simulink model "simulink_group8"  (R2020a)
settings: Solver=FixedStepAuto  StartTime=0.0  StopTime=10.0  FixedStep=1e-3  RelTol=1e-3  EnableMultiTasking=on
undefined symbols (not defined in the file): D0, D1, D10, D11, D12, D13, D2, D3, D4, D5, D6, D7, D8, D9, PTA0, PTA1, PTA2, PTB23, PTB9, PTC16, PTC17, PTC2, PTC3, PTC4, PTD0, PTD1, PTD2, PTD3
libraries: frdmk64flib x14
settings Model: ExtModeTrigDuration=5  Creator=namby  LastModifiedBy=namby
settings OptimizationCC: EnhancedBackFolding=on  PassReuseOutputArgsAs=Individual arguments  ZeroExternalMemoryAtStartup=off  ZeroInternalMemoryAtStartup=off  MaxStackSize=64  OptimizeBlockOrder=speed  DifferentSizesBufferReuse=on  OptimizationCustomize=off  EfficientTunableParamExpr=on
settings DebuggingCC: ParameterTunabilityLossMsg=error
settings HardwareCC: ProdBitPerPointer=32  ProdBitPerSizeT=32  ProdBitPerPtrDiffT=32  ProdLargestAtomicInteger=Long  ProdLargestAtomicFloat=Double  ProdWordSize=32  ProdHWDeviceType=ARM Compatible->ARM Cortex
settings SFSimCC: MATLABDynamicMemAlloc=off
settings RTWCC: SystemTargetFile=ert.tlc  HardwareBoard=NXP FRDM-K64F  TemplateMakefile=ert_default_tmf  Toolchain=GNU Tools for ARM Embedded Processors
settings CodeAppCC: ForceParamTrailComments=on  IgnoreCustomStorageClasses=off  OperatorAnnotations=on  SimulinkDataObjDesc=on  SFDataObjDesc=on  InsertBlockDesc=on

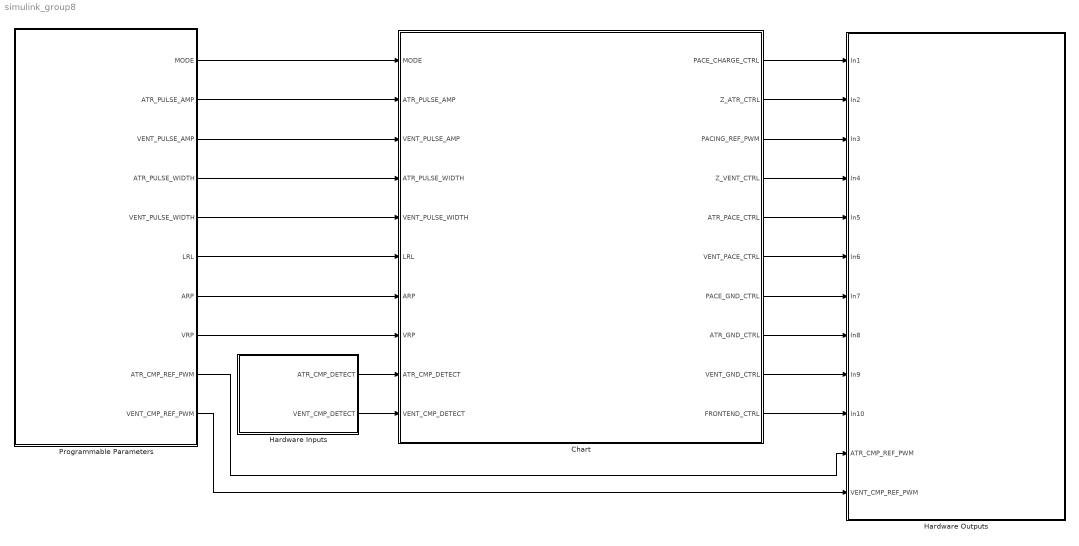
== system simulink_group8 ==
  Chart : Stateflow chart  TreatAsAtomicUnit=on
  Hardware Inputs : Subsystem
  Hardware Outputs : Subsystem
  Programmable Parameters : Subsystem
  wires:
  Programmable Parameters/1(MODE) -> Chart/1(MODE)
  Programmable Parameters/2(ATR_PULSE_AMP) -> Chart/2(ATR_PULSE_AMP)
  Programmable Parameters/3(VENT_PULSE_AMP) -> Chart/3(VENT_PULSE_AMP)
  Programmable Parameters/4(ATR_PULSE_WIDTH) -> Chart/4(ATR_PULSE_WIDTH)
  Programmable Parameters/5(VENT_PULSE_WIDTH) -> Chart/5(VENT_PULSE_WIDTH)
  Programmable Parameters/6(LRL) -> Chart/6(LRL)
  Programmable Parameters/7(ARP) -> Chart/7(ARP)
  Programmable Parameters/8(VRP) -> Chart/8(VRP)
  Hardware Inputs/1(ATR_CMP_DETECT) -> Chart/9(ATR_CMP_DETECT)
  Hardware Inputs/2(VENT_CMP_DETECT) -> Chart/10(VENT_CMP_DETECT)
  Chart/1(PACE_CHARGE_CTRL) -> Hardware Outputs/1(In1)
  Chart/2(Z_ATR_CTRL) -> Hardware Outputs/2(In2)
  Chart/3(PACING_REF_PWM) -> Hardware Outputs/3(In3)
  Chart/4(Z_VENT_CTRL) -> Hardware Outputs/4(In4)
  Chart/5(ATR_PACE_CTRL) -> Hardware Outputs/5(In5)
  Chart/6(VENT_PACE_CTRL) -> Hardware Outputs/6(In6)
  Chart/7(PACE_GND_CTRL) -> Hardware Outputs/7(In7)
  Chart/8(ATR_GND_CTRL) -> Hardware Outputs/8(In8)
  Chart/9(VENT_GND_CTRL) -> Hardware Outputs/9(In9)
  Chart/10(FRONTEND_CTRL) -> Hardware Outputs/10(In10)
  Programmable Parameters/9(ATR_CMP_REF_PWM) -> Hardware Outputs/11(ATR_CMP_REF_PWM)
  Programmable Parameters/10(VENT_CMP_REF_PWM) -> Hardware Outputs/12(VENT_CMP_REF_PWM)

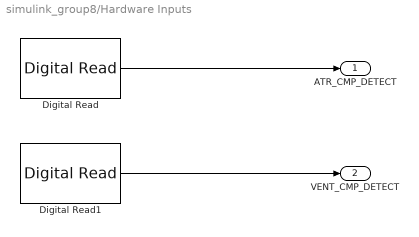
== system simulink_group8/Hardware Inputs ==
  Digital Read : frdmk64flib/Digital Read  Whichpin=PTC16 (D0)  SampleTime=-1
  Digital Read1 : frdmk64flib/Digital Read  Whichpin=PTC17 (D1)  SampleTime=-1
  ATR_CMP_DETECT : Outport
  VENT_CMP_DETECT : Outport  Port=2
  wires:
  Digital Read/1 -> ATR_CMP_DETECT/1
  Digital Read1/1 -> VENT_CMP_DETECT/1

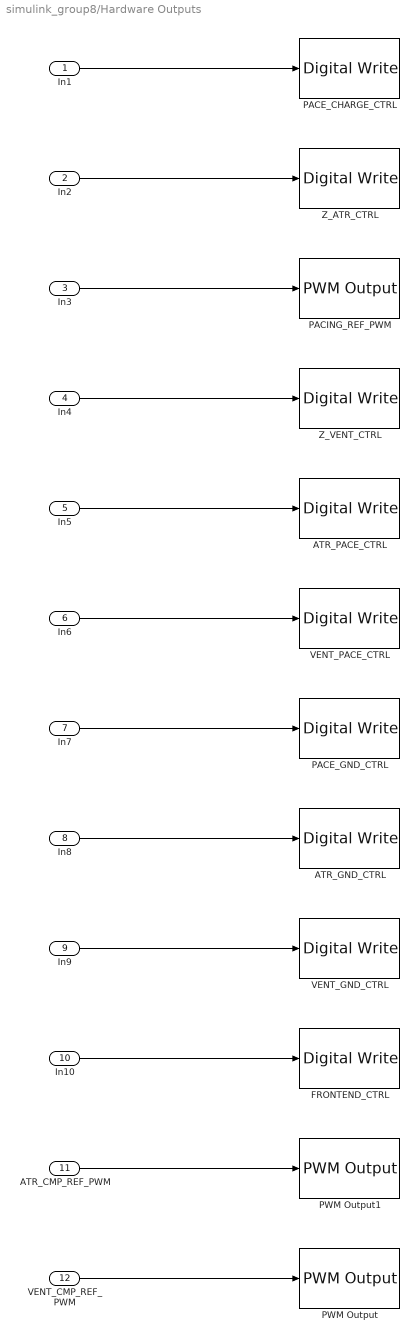
== system simulink_group8/Hardware Outputs ==
  In1 : Inport
  In2 : Inport  Port=2
  In3 : Inport  Port=3
  In4 : Inport  Port=4
  In5 : Inport  Port=5
  In6 : Inport  Port=6
  In7 : Inport  Port=7
  In8 : Inport  Port=8
  In9 : Inport  Port=9
  In10 : Inport  Port=10
  ATR_CMP_REF_PWM : Inport  Port=11
  VENT_CMP_REF_PWM : Inport  Port=12
  ATR_GND_CTRL : frdmk64flib/Digital Write  Whichpin=PTD2 (D11)
  ATR_PACE_CTRL : frdmk64flib/Digital Write  Whichpin=PTA0 (D8)
  FRONTEND_CTRL : frdmk64flib/Digital Write  Whichpin=PTD1 (D13)
  PACE_CHARGE_CTRL : frdmk64flib/Digital Write  Whichpin=PTB9 (D2)
  PACE_GND_CTRL : frdmk64flib/Digital Write  Whichpin=PTD0 (D10)
  PACING_REF_PWM : frdmk64flib/PWM Output  Whichpin=PTA2 (D5)  InitialFrequency=2000  InitialDutyCycle=0
  PWM Output : frdmk64flib/PWM Output  Whichpin=PTA1 (D3)  InitialFrequency=2000  InitialDutyCycle=0
  PWM Output1 : frdmk64flib/PWM Output  Whichpin=PTC2 (D6)  InitialFrequency=2000  InitialDutyCycle=0
  VENT_GND_CTRL : frdmk64flib/Digital Write  Whichpin=PTD3 (D12)
  VENT_PACE_CTRL : frdmk64flib/Digital Write  Whichpin=PTC4 (D9)
  Z_ATR_CTRL : frdmk64flib/Digital Write  Whichpin=PTB23 (D4)
  Z_VENT_CTRL : frdmk64flib/Digital Write  Whichpin=PTC3 (D7)
  wires:
  In1/1 -> PACE_CHARGE_CTRL/1
  In2/1 -> Z_ATR_CTRL/1
  In3/1 -> PACING_REF_PWM/1
  In4/1 -> Z_VENT_CTRL/1
  In5/1 -> ATR_PACE_CTRL/1
  In6/1 -> VENT_PACE_CTRL/1
  In8/1 -> ATR_GND_CTRL/1
  In7/1 -> PACE_GND_CTRL/1
  In10/1 -> FRONTEND_CTRL/1
  In9/1 -> VENT_GND_CTRL/1
  ATR_CMP_REF_PWM/1 -> PWM Output1/1
  VENT_CMP_REF_PWM/1 -> PWM Output/1

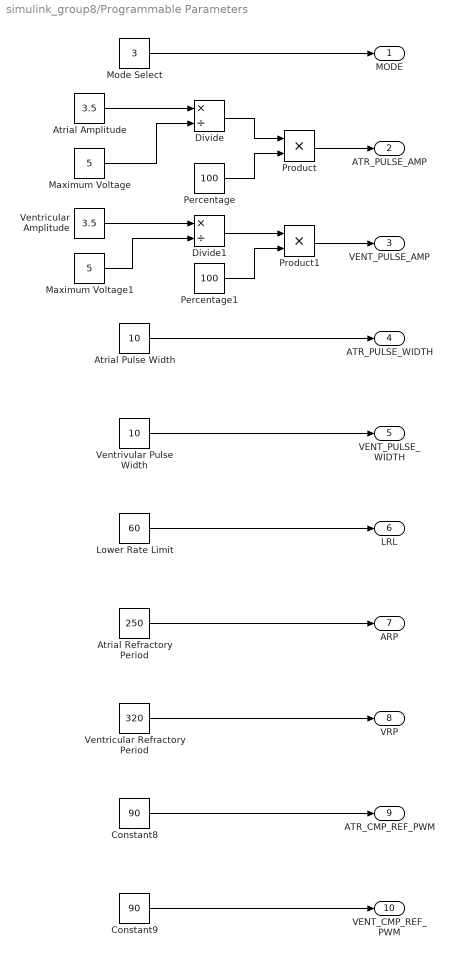
== system simulink_group8/Programmable Parameters ==
  Atrial Amplitude : Constant  Value=3.5
  Atrial Pulse Width : Constant  Value=10
  Atrial Refractory Period : Constant  Value=250
  Constant8 : Constant  Value=90
  Constant9 : Constant  Value=90
  Divide : Product  Inputs=*/
  Divide1 : Product  Inputs=*/
  Lower Rate Limit : Constant  Value=60
  Maximum Voltage : Constant  Value=5
  Maximum Voltage1 : Constant  Value=5
  Mode Select : Constant  Value=3
  Percentage : Constant  Value=100
  Percentage1 : Constant  Value=100
  Product : Product
  Product1 : Product
  Ventricular Amplitude : Constant  Value=3.5
  Ventricular Refractory Period : Constant  Value=320
  Ventrivular Pulse Width : Constant  Value=10
  MODE : Outport
  ATR_PULSE_AMP : Outport  Port=2
  VENT_PULSE_AMP : Outport  Port=3
  ATR_PULSE_WIDTH : Outport  Port=4
  VENT_PULSE_WIDTH : Outport  Port=5
  LRL : Outport  Port=6
  ARP : Outport  Port=7
  VRP : Outport  Port=8
  ATR_CMP_REF_PWM : Outport  Port=9
  VENT_CMP_REF_PWM : Outport  Port=10
  wires:
  Mode Select/1 -> MODE/1
  Ventrivular Pulse Width/1 -> VENT_PULSE_WIDTH/1
  Atrial Pulse Width/1 -> ATR_PULSE_WIDTH/1
  Lower Rate Limit/1 -> LRL/1
  Atrial Refractory Period/1 -> ARP/1
  Ventricular Refractory Period/1 -> VRP/1
  Constant8/1 -> ATR_CMP_REF_PWM/1
  Constant9/1 -> VENT_CMP_REF_PWM/1
  Atrial Amplitude/1 -> Divide/1
  Maximum Voltage/1 -> Divide/2
  Percentage/1 -> Product/2
  Divide/1 -> Product/1
  Product/1 -> ATR_PULSE_AMP/1
  Percentage1/1 -> Product1/2
  Ventricular Amplitude/1 -> Divide1/1
  Divide1/1 -> Product1/1
  Maximum Voltage1/1 -> Divide1/2
  Product1/1 -> VENT_PULSE_AMP/1

== stateflow chart simulink_group8/Chart ==
  state DEFAULT_STATE
    FRONTEND_CTRL = 0
  state AOO
    state STATE_2
      %Atrium Pacing
      PACE_CHARGE_CTRL = 0
      PACE_GND_CTRL = 1
      ATR_PACE_CTRL = 1
      ATR_GND_CTRL = 0
      Z_ATR_CTRL = 0
      Z_VENT_CTRL = 0
      VENT_GND_CTRL = 0
      VENT_PACE_CTRL = 0
    state STATE_1
      %Charging primary capacitor (C22)
      ATR_PACE_CTRL = 0
      VENT_PACE_CTRL = 0
      PACING_REF_PWM = ATR_PULSE_AMP
      PACE_CHARGE_CTRL = 1
      %
      %Discharging blocking capacitor (C21)
      PACE_GND_CTRL = 1
      VENT_PACE_CTRL = 0
      Z_ATR_CTRL = 0
      Z_VENT_CTRL = 0
      ATR_PACE_CTRL = 0
      ATR_GND_CTRL = 1
      VENT_GND_CTRL = 0
    (default) -> AOO.STATE_1
    AOO.STATE_1 -> AOO.STATE_2 [order 1] : [after((60000/LRL) - ATR_PULSE_WIDTH, msec)]
    AOO.STATE_2 -> AOO.STATE_1 : [after(ATR_PULSE_WIDTH, msec)]
  state VOO
    state STATE_2
      %Ventricular Pacing
      PACE_CHARGE_CTRL = 0
      PACE_GND_CTRL = 1
      ATR_PACE_CTRL = 0
      ATR_GND_CTRL = 0
      Z_ATR_CTRL = 0
      Z_VENT_CTRL = 0
      VENT_GND_CTRL = 0
      VENT_PACE_CTRL = 1
    state STATE_1
      %Charging primary capacitor (C22)
      ATR_PACE_CTRL = 0
      VENT_PACE_CTRL = 0
      PACING_REF_PWM = VENT_PULSE_AMP
      PACE_CHARGE_CTRL = 1
      %
      %Discharging blocking capacitor (C21)
      PACE_GND_CTRL = 1
      VENT_PACE_CTRL = 0
      Z_ATR_CTRL = 0
      Z_VENT_CTRL = 0
      ATR_PACE_CTRL = 0
      ATR_GND_CTRL = 0
      VENT_GND_CTRL = 1
    (default) -> VOO.STATE_1
    VOO.STATE_1 -> VOO.STATE_2 [order 1] : [after((60000/LRL) - VENT_PULSE_WIDTH, msec)]
    VOO.STATE_2 -> VOO.STATE_1 : [after(VENT_PULSE_WIDTH, msec)]
  state AAI
    state ATR_SENSE
    state STATE_1
      %Enable sensing
      FRONTEND_CTRL = 1
      %
      %Charging primary capacitor (C22)
      ATR_PACE_CTRL = 0
      VENT_PACE_CTRL = 0
      PACING_REF_PWM = ATR_PULSE_AMP
      PACE_CHARGE_CTRL = 1
      %
      %Discharging blocking capacitor (C21)
      PACE_GND_CTRL = 1
      VENT_PACE_CTRL = 0
      Z_ATR_CTRL = 0
      Z_VENT_CTRL = 0
      ATR_PACE_CTRL = 0
      ATR_GND_CTRL = 1
      VENT_GND_CTRL = 0
    state STATE_2
      %Atrium Pacing
      PACE_CHARGE_CTRL = 0
      PACE_GND_CTRL = 1
      ATR_PACE_CTRL = 1
      ATR_GND_CTRL = 0
      Z_ATR_CTRL = 0
      Z_VENT_CTRL = 0
      VENT_GND_CTRL = 0
      VENT_PACE_CTRL = 0
    ATR_SENSE -> AAI.STATE_2 [order 2] : after((60000/LRL) - ATR_PULSE_WIDTH - ARP, msec)[ATR_CMP_DETECT == 0]
    AAI.STATE_1 -> ATR_SENSE [order 1] : [after(ARP, msec)]
    ATR_SENSE -> AAI.STATE_1 [order 1] : [ATR_CMP_DETECT == 1]
    (default) -> AAI.STATE_1
    AAI.STATE_2 -> AAI.STATE_1 : [after(ATR_PULSE_WIDTH, msec)]
  state VVI
    state VENT_SENSE
    state STATE_2
      %Ventricular Pacing
      PACE_CHARGE_CTRL = 0
      PACE_GND_CTRL = 1
      ATR_PACE_CTRL = 0
      ATR_GND_CTRL = 0
      Z_ATR_CTRL = 0
      Z_VENT_CTRL = 0
      VENT_GND_CTRL = 0
      VENT_PACE_CTRL = 1
    state STATE_1
      %Enable Sensing
      FRONTEND_CTRL = 1
      %
      %Charging primary capacitor (C22)
      ATR_PACE_CTRL = 0
      VENT_PACE_CTRL = 0
      PACING_REF_PWM = VENT_PULSE_AMP
      PACE_CHARGE_CTRL = 1
      %
      %Discharging blocking capacitor (C21)
      PACE_GND_CTRL = 1
      VENT_PACE_CTRL = 0
      Z_ATR_CTRL = 0
      Z_VENT_CTRL = 0
      ATR_PACE_CTRL = 0
      ATR_GND_CTRL = 0
      VENT_GND_CTRL = 1
    VENT_SENSE -> VVI.STATE_2 [order 1] : after((60000/LRL) - VENT_PULSE_WIDTH - VRP, msec)[VENT_CMP_DETECT == 0]
    VVI.STATE_1 -> VENT_SENSE [order 1] : [after(VRP, msec)]
    VENT_SENSE -> VVI.STATE_1 [order 2] : [VENT_CMP_DETECT==1]
    (default) -> VVI.STATE_1
    VVI.STATE_2 -> VVI.STATE_1 : [after(VENT_PULSE_WIDTH, msec)]
  VOO.STATE_1 -> DEFAULT_STATE [order 2] : [MODE~=2]
  AAI.STATE_1 -> DEFAULT_STATE [order 2] : [MODE~=3]
  AOO.STATE_1 -> DEFAULT_STATE [order 2] : [MODE~=1]
  VVI.STATE_1 -> DEFAULT_STATE [order 2] : [MODE~=4]
  DEFAULT_STATE -> AAI.STATE_1 [order 3] : [MODE==3]
  DEFAULT_STATE -> VVI.STATE_1 [order 4] : [MODE==4]
  DEFAULT_STATE -> VOO.STATE_1 [order 2] : [MODE==2]
  DEFAULT_STATE -> AOO.STATE_1 [order 1] : [MODE==1]
  (default) -> DEFAULT_STATE
  data: PACE_CHARGE_CTRL output; Z_ATR_CTRL output; PACING_REF_PWM output; Z_VENT_CTRL output; ATR_PACE_CTRL output; VENT_PACE_CTRL output; PACE_GND_CTRL output; ATR_GND_CTRL output; VENT_GND_CTRL output; FRONTEND_CTRL output; MODE input; ATR_PULSE_AMP input; VENT_PULSE_AMP input; ATR_PULSE_WIDTH input; VENT_PULSE_WIDTH input; LRL input; ARP input; VRP input; ATR_CMP_DETECT input; VENT_CMP_DETECT input
